simulink library "ECO_TestLibs"  (R2018a)
settings: Solver=ode45  StartTime=0.0  StopTime=10.0  RelTol=1e-3  EnableMultiTasking=on
undefined symbols (not defined in the file or in its folder): h, km
libraries: CoderSF_BSW_Libs x643, $bdroot x217, SF_CanService_Libs x60, simulink x12
(part 6 of 7)

== system ECO_TestLibs/LINASlave/Rx/Subsystem2 ==
  In1 : Inport
  Enable : EnablePort
  1 : Constant  Value=0  OutDataTypeStr=Inherit: Inherit via back propagation
  2 : Constant  Value=0  OutDataTypeStr=Inherit: Inherit via back propagation
  3 : Constant  Value=hex2dec('212')  OutDataTypeStr=Inherit: Inherit via back propagation
  4 : Constant  Value=8  OutDataTypeStr=Inherit: Inherit via back propagation
  Demux : Demux  Outputs=3
  Transmit CAN Message : CoderSF_BSW_Libs/CAN/Transmit CAN Message  channel=CAN_C  tasktimeIndex=Task_Inherit
      settings: SourceProductName=EcoCoder Blocks
  Vector Concatenate : Concatenate  NumInputs=8
  Write Measurement : CoderSF_BSW_Libs/Calibration & Measurement/Write Measurement  variable_name=LIN_Rx2  variable_value=0  variable_type=uint8  numD=3  unitStr=""  descStr=""
      settings: AttributesFormatString=type:%<variable_type> Dimensions:%<numD>  SourceProductName=EcoCoder Blocks
  cntValue : Subsystem
  wires:
  In1/1 -> Demux/1, Write Measurement/1
  3/1 -> Transmit CAN Message/3
  4/1 -> Transmit CAN Message/4
  2/1 -> Transmit CAN Message/2
  1/1 -> Transmit CAN Message/1
  Demux/2 -> Vector Concatenate/2
  Demux/1 -> Vector Concatenate/1
  Demux/3 -> Vector Concatenate/3
  Vector Concatenate/1 -> Transmit CAN Message/5
  cntValue/1(Out1) -> Vector Concatenate/4
  cntValue/2(Out2) -> Vector Concatenate/5
  cntValue/3(Out3) -> Vector Concatenate/6
  cntValue/4(Out4) -> Vector Concatenate/7
  cntValue/5(Out5) -> Vector Concatenate/8

== system ECO_TestLibs/LINASlave/Transmit/Tx ==
  Constant : Constant  OutDataTypeStr=uint8
  Constant1 : Constant  Value=2  OutDataTypeStr=uint8
  Data Type Conversion : DataTypeConversion
  Data Type Conversion1 : DataTypeConversion
  Delay : simulink/Discrete/Integer Delay  NumDelays=1  vinit=0  samptime=-1
      settings: SourceProductName=Simulink  SourceProductBaseCode=SL
  Delay1 : simulink/Discrete/Integer Delay  NumDelays=1  vinit=0  samptime=-1
      settings: SourceProductName=Simulink  SourceProductBaseCode=SL
  LIN Transmit Data2 : CoderSF_BSW_Libs/LIN/LIN Transmit Data  channel=LIN_A  Frame_Id=hex2dec('4')  Frame_Len=8  Frame_Dir=MasterReceive  Frame_CCS=Enhanced  Task_TimeIdx=Task_Inherit
      settings: SourceProductName=EcoCoder Blocks
  LIN Transmit Data3 : CoderSF_BSW_Libs/LIN/LIN Transmit Data  channel=LIN_A  Frame_Id=hex2dec('5')  Frame_Len=8  Frame_Dir=MasterReceive  Frame_CCS=Enhanced  Task_TimeIdx=Task_Inherit
      settings: SourceProductName=EcoCoder Blocks
  Mux : Mux  Inputs=8
  Mux1 : Mux  Inputs=8
  Sum : Sum  Inputs=|++
  Sum1 : Sum  Inputs=|++
  Write and Read Measurement : CoderSF_BSW_Libs/Calibration & Measurement/Write and Read Measurement  variable_name=LIN_ID4_SendData  variable_value=0  variable_type=uint8  numD=8  unitStr=""  descStr=""
      settings: AttributesFormatString=type:%<variable_type> Dimensions:%<numD>  SourceProductName=EcoCoder Blocks
  Write and Read Measurement1 : CoderSF_BSW_Libs/Calibration & Measurement/Write and Read Measurement  variable_name=LIN_ID5_SendData  variable_value=0  variable_type=uint8  numD=8  unitStr=""  descStr=""
      settings: AttributesFormatString=type:%<variable_type> Dimensions:%<numD>  SourceProductName=EcoCoder Blocks
  wires:
  Mux/1 -> Data Type Conversion/1
  Mux1/1 -> Data Type Conversion1/1
  Sum/1 -> Delay/1
  Constant/1 -> Sum/2
  Delay1/1 -> Sum1/1, Mux1/8, Mux1/7, Mux1/6, Mux1/5, Mux1/4, Mux1/3, Mux1/2, Mux1/1
  Sum1/1 -> Delay1/1
  Constant1/1 -> Sum1/2
  Write and Read Measurement/1 -> LIN Transmit Data2/1
  Data Type Conversion/1 -> Write and Read Measurement/1
  Delay/1 -> Mux/8, Mux/7, Mux/6, Mux/5, Mux/4, Mux/3, Mux/2, Mux/1, Sum/1
  Data Type Conversion1/1 -> Write and Read Measurement1/1
  Write and Read Measurement1/1 -> LIN Transmit Data3/1

== system ECO_TestLibs/TAF_CANA/Connected/Subsystem ==
  In1 : Inport
  In2 : Inport  Port=2
  In3 : Inport  Port=3
  In4 : Inport  Port=4
  In5 : Inport  Port=5
  In6 : Inport  Port=6
  In7 : Inport  Port=7
  In8 : Inport  Port=8
  Enable : EnablePort
  Plus1_{0..7} (8 alike) : $bdroot/Plus1_0
  Send Fixed-Point CAN Message : SF_CanService_Libs/Send Fixed-Point CAN Message  typeCAN=Connected  channel=CAN_A  mEn=off  msgInfo=TAF_CAN_new  msgIterm=CAN0x402  msgItermStore=CAN0x402  motoBit=off  flgNoFixed=off  tSample=Task_Inherit  modeCode=Parameterless
  wires:
  Plus1_4/1 -> Send Fixed-Point CAN Message/5
  Plus1_7/1 -> Send Fixed-Point CAN Message/8
  Plus1_6/1 -> Send Fixed-Point CAN Message/7
  Plus1_5/1 -> Send Fixed-Point CAN Message/6
  Plus1_3/1 -> Send Fixed-Point CAN Message/4
  Plus1_2/1 -> Send Fixed-Point CAN Message/3
  Plus1_1/1 -> Send Fixed-Point CAN Message/2
  Plus1_0/1 -> Send Fixed-Point CAN Message/1
  In7/1 -> Plus1_6/1
  In6/1 -> Plus1_5/1
  In8/1 -> Plus1_7/1
  In2/1 -> Plus1_1/1
  In3/1 -> Plus1_2/1
  In1/1 -> Plus1_0/1
  In5/1 -> Plus1_4/1
  In4/1 -> Plus1_3/1

== system ECO_TestLibs/TAF_CANA/Connected/Subsystem1 ==
  In1 : Inport
  In2 : Inport  Port=2
  In3 : Inport  Port=3
  In4 : Inport  Port=4
  In5 : Inport  Port=5
  In6 : Inport  Port=6
  In7 : Inport  Port=7
  In8 : Inport  Port=8
  Enable : EnablePort
  Mux : Mux  Inputs=8
  Plus1_0 : $bdroot/Plus1_0
  Plus1_{1..7} (7 alike) : $bdroot/Plus2_0
  Plus2_0 : $bdroot/Plus2_0
  Send CAN Data : CoderSF_BSW_Libs/CAN/Send CAN Data  channel=CAN_A  txlen=8  txid=hex2dec('412')  frametype=Extended(29-bit ID)  showerror=off
      settings: SourceProductName=EcoCoder Blocks
  Send CAN Message : SF_CanService_Libs/Send CAN Message   typeCAN=Connected  channel=CAN_A  mEn=off  msgInfo=TAF_CAN_new  msgIterm=CAN0x402x  msgItermStore=CAN0x402x  motoBit=off  flgNoFixed=off  tSample=Task_Inherit  modeCode=Parameterless
  wires:
  Plus1_0/1 -> Send CAN Data/1
  Mux/1 -> Plus1_0/1
  In4/1 -> Plus1_3/1
  In5/1 -> Plus1_4/1
  In1/1 -> Plus2_0/1
  In3/1 -> Plus1_2/1
  In2/1 -> Plus1_1/1
  In8/1 -> Plus1_7/1
  In6/1 -> Plus1_5/1
  In7/1 -> Plus1_6/1
  Plus2_0/1 -> Send CAN Message/1, Mux/1
  Plus1_1/1 -> Send CAN Message/2, Mux/2
  Plus1_2/1 -> Send CAN Message/3, Mux/3
  Plus1_3/1 -> Send CAN Message/4, Mux/4
  Plus1_5/1 -> Send CAN Message/6, Mux/6
  Plus1_6/1 -> Send CAN Message/7, Mux/7
  Plus1_7/1 -> Send CAN Message/8, Mux/8
  Plus1_4/1 -> Send CAN Message/5, Mux/5

== system ECO_TestLibs/TAF_CANA/Disconnected/Subsystem ==
  In1 : Inport
  In2 : Inport  Port=2
  In3 : Inport  Port=3
  In4 : Inport  Port=4
  In5 : Inport  Port=5
  In6 : Inport  Port=6
  In7 : Inport  Port=7
  In8 : Inport  Port=8
  Enable : EnablePort
  Plus1_{0..7} (8 alike) : $bdroot/Plus1_0
  Send Fixed-Point CAN Message : SF_CanService_Libs/Send Fixed-Point CAN Message  typeCAN=Disconnected  channel=CAN_A  mEn=off  msgInfo=TAF_CAN_new  msgIterm=CAN0x401  msgItermStore=CAN0x401  motoBit=off  flgNoFixed=off  tSample=Task_Inherit  modeCode=Parameterless
  Transmit CAN Message : CoderSF_BSW_Libs/CAN/Transmit CAN Message  channel=CAN_A  tasktimeIndex=Task_Inherit
      settings: SourceProductName=EcoCoder Blocks
  wires:
  In4/1 -> Plus1_3/1
  In5/1 -> Plus1_4/1
  In1/1 -> Plus1_0/1
  In3/1 -> Plus1_2/1
  In2/1 -> Plus1_1/1
  In8/1 -> Plus1_7/1
  In6/1 -> Plus1_5/1
  In7/1 -> Plus1_6/1
  Plus1_0/1 -> Send Fixed-Point CAN Message/1
  Plus1_1/1 -> Send Fixed-Point CAN Message/2
  Plus1_2/1 -> Send Fixed-Point CAN Message/3
  Plus1_3/1 -> Send Fixed-Point CAN Message/4
  Plus1_5/1 -> Send Fixed-Point CAN Message/6
  Plus1_6/1 -> Send Fixed-Point CAN Message/7
  Plus1_7/1 -> Send Fixed-Point CAN Message/8
  Plus1_4/1 -> Send Fixed-Point CAN Message/5
  Send Fixed-Point CAN Message/4 -> Transmit CAN Message/4
  Send Fixed-Point CAN Message/5 -> Transmit CAN Message/5
  Send Fixed-Point CAN Message/1 -> Transmit CAN Message/1
  Send Fixed-Point CAN Message/2 -> Transmit CAN Message/2
  Send Fixed-Point CAN Message/3 -> Transmit CAN Message/3

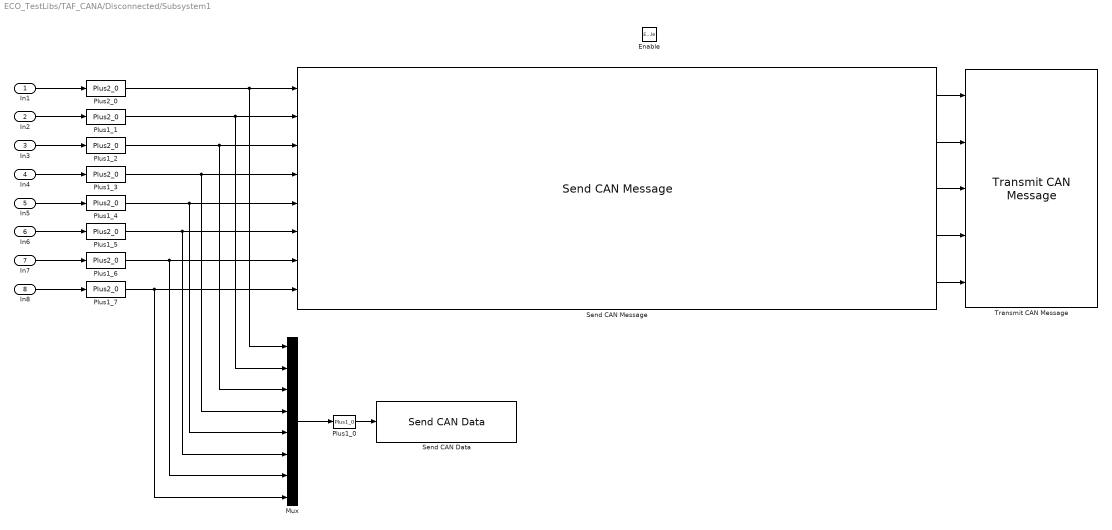
== system ECO_TestLibs/TAF_CANA/Disconnected/Subsystem1 ==
  In1 : Inport
  In2 : Inport  Port=2
  In3 : Inport  Port=3
  In4 : Inport  Port=4
  In5 : Inport  Port=5
  In6 : Inport  Port=6
  In7 : Inport  Port=7
  In8 : Inport  Port=8
  Enable : EnablePort
  Mux : Mux  Inputs=8
  Plus1_0 : $bdroot/Plus1_0
  Plus1_{1..7} (7 alike) : $bdroot/Plus2_0
  Plus2_0 : $bdroot/Plus2_0
  Send CAN Data : CoderSF_BSW_Libs/CAN/Send CAN Data  channel=CAN_A  txlen=8  txid=hex2dec('411')  frametype=Extended(29-bit ID)  showerror=off
      settings: SourceProductName=EcoCoder Blocks
  Send CAN Message : SF_CanService_Libs/Send CAN Message   typeCAN=Disconnected  channel=CAN_A  mEn=off  msgInfo=TAF_CAN_new  msgIterm=CAN0x401x  msgItermStore=CAN0x401x  motoBit=off  flgNoFixed=off  tSample=Task_Inherit  modeCode=Parameterless
  Transmit CAN Message : CoderSF_BSW_Libs/CAN/Transmit CAN Message  channel=CAN_A  tasktimeIndex=Task_Inherit
      settings: SourceProductName=EcoCoder Blocks
  wires:
  Plus1_4/1 -> Mux/5, Send CAN Message/5
  Plus1_7/1 -> Mux/8, Send CAN Message/8
  Plus1_6/1 -> Mux/7, Send CAN Message/7
  Plus1_5/1 -> Mux/6, Send CAN Message/6
  Plus1_3/1 -> Mux/4, Send CAN Message/4
  Plus1_2/1 -> Mux/3, Send CAN Message/3
  Plus1_1/1 -> Mux/2, Send CAN Message/2
  Plus2_0/1 -> Mux/1, Send CAN Message/1
  In7/1 -> Plus1_6/1
  In6/1 -> Plus1_5/1
  In8/1 -> Plus1_7/1
  In2/1 -> Plus1_1/1
  In3/1 -> Plus1_2/1
  In1/1 -> Plus2_0/1
  In5/1 -> Plus1_4/1
  In4/1 -> Plus1_3/1
  Mux/1 -> Plus1_0/1
  Plus1_0/1 -> Send CAN Data/1
  Send CAN Message/1 -> Transmit CAN Message/1
  Send CAN Message/5 -> Transmit CAN Message/5
  Send CAN Message/4 -> Transmit CAN Message/4
  Send CAN Message/2 -> Transmit CAN Message/2
  Send CAN Message/3 -> Transmit CAN Message/3

== system ECO_TestLibs/TAF_CANB/Connected/Subsystem1 ==
  In1 : Inport
  In2 : Inport  Port=2
  In3 : Inport  Port=3
  In4 : Inport  Port=4
  In5 : Inport  Port=5
  In6 : Inport  Port=6
  In7 : Inport  Port=7
  In8 : Inport  Port=8
  Enable : EnablePort
  Plus1_{0..7} (8 alike) : $bdroot/Plus1_0
  Send Fixed-Point CAN Message : SF_CanService_Libs/Send Fixed-Point CAN Message  typeCAN=Connected  channel=CAN_B  mEn=off  msgInfo=TAF_CAN_new  msgIterm=CAN0x404  msgItermStore=CAN0x404  motoBit=off  flgNoFixed=off  tSample=Task_Inherit  modeCode=Parameterless
  wires:
  Plus1_4/1 -> Send Fixed-Point CAN Message/5
  Plus1_7/1 -> Send Fixed-Point CAN Message/8
  Plus1_6/1 -> Send Fixed-Point CAN Message/7
  Plus1_5/1 -> Send Fixed-Point CAN Message/6
  Plus1_3/1 -> Send Fixed-Point CAN Message/4
  Plus1_2/1 -> Send Fixed-Point CAN Message/3
  Plus1_1/1 -> Send Fixed-Point CAN Message/2
  Plus1_0/1 -> Send Fixed-Point CAN Message/1
  In7/1 -> Plus1_6/1
  In6/1 -> Plus1_5/1
  In8/1 -> Plus1_7/1
  In2/1 -> Plus1_1/1
  In3/1 -> Plus1_2/1
  In1/1 -> Plus1_0/1
  In5/1 -> Plus1_4/1
  In4/1 -> Plus1_3/1

== system ECO_TestLibs/TAF_CANB/Connected/Subsystem5 ==
  In1 : Inport
  In2 : Inport  Port=2
  In3 : Inport  Port=3
  In4 : Inport  Port=4
  In5 : Inport  Port=5
  In6 : Inport  Port=6
  In7 : Inport  Port=7
  In8 : Inport  Port=8
  Enable : EnablePort
  Mux : Mux  Inputs=8
  Plus1_0 : $bdroot/Plus1_0
  Plus1_{1..7} (7 alike) : $bdroot/Plus2_0
  Plus2_0 : $bdroot/Plus2_0
  Send CAN Data : CoderSF_BSW_Libs/CAN/Send CAN Data  channel=CAN_B  txlen=8  txid=hex2dec('414')  frametype=Extended(29-bit ID)  showerror=off
      settings: SourceProductName=EcoCoder Blocks
  Send CAN Message : SF_CanService_Libs/Send CAN Message   typeCAN=Connected  channel=CAN_B  mEn=off  msgInfo=TAF_CAN_new  msgIterm=CAN0x404x  msgItermStore=CAN0x404x  motoBit=off  flgNoFixed=off  tSample=Task_Inherit  modeCode=Parameterless
  wires:
  Plus1_0/1 -> Send CAN Data/1
  Mux/1 -> Plus1_0/1
  In4/1 -> Plus1_3/1
  In5/1 -> Plus1_4/1
  In1/1 -> Plus2_0/1
  In3/1 -> Plus1_2/1
  In2/1 -> Plus1_1/1
  In8/1 -> Plus1_7/1
  In6/1 -> Plus1_5/1
  In7/1 -> Plus1_6/1
  Plus2_0/1 -> Send CAN Message/1, Mux/1
  Plus1_1/1 -> Send CAN Message/2, Mux/2
  Plus1_2/1 -> Send CAN Message/3, Mux/3
  Plus1_3/1 -> Send CAN Message/4, Mux/4
  Plus1_5/1 -> Send CAN Message/6, Mux/6
  Plus1_6/1 -> Send CAN Message/7, Mux/7
  Plus1_7/1 -> Send CAN Message/8, Mux/8
  Plus1_4/1 -> Send CAN Message/5, Mux/5

== system ECO_TestLibs/TAF_CANB/Disconnected/Subsystem1 ==
  In1 : Inport
  In2 : Inport  Port=2
  In3 : Inport  Port=3
  In4 : Inport  Port=4
  In5 : Inport  Port=5
  In6 : Inport  Port=6
  In7 : Inport  Port=7
  In8 : Inport  Port=8
  Enable : EnablePort
  Plus1_{0..7} (8 alike) : $bdroot/Plus1_0
  Send Fixed-Point CAN Message : SF_CanService_Libs/Send Fixed-Point CAN Message  typeCAN=Disconnected  channel=CAN_B  mEn=off  msgInfo=TAF_CAN_new  msgIterm=CAN0x403  msgItermStore=CAN0x403  motoBit=off  flgNoFixed=off  tSample=Task_Inherit  modeCode=Parameterless
  Transmit CAN Message : CoderSF_BSW_Libs/CAN/Transmit CAN Message  channel=CAN_B  tasktimeIndex=Task_Inherit
      settings: SourceProductName=EcoCoder Blocks
  wires:
  In4/1 -> Plus1_3/1
  In5/1 -> Plus1_4/1
  In1/1 -> Plus1_0/1
  In3/1 -> Plus1_2/1
  In2/1 -> Plus1_1/1
  In8/1 -> Plus1_7/1
  In6/1 -> Plus1_5/1
  In7/1 -> Plus1_6/1
  Plus1_0/1 -> Send Fixed-Point CAN Message/1
  Plus1_1/1 -> Send Fixed-Point CAN Message/2
  Plus1_2/1 -> Send Fixed-Point CAN Message/3
  Plus1_3/1 -> Send Fixed-Point CAN Message/4
  Plus1_5/1 -> Send Fixed-Point CAN Message/6
  Plus1_6/1 -> Send Fixed-Point CAN Message/7
  Plus1_7/1 -> Send Fixed-Point CAN Message/8
  Plus1_4/1 -> Send Fixed-Point CAN Message/5
  Send Fixed-Point CAN Message/3 -> Transmit CAN Message/3
  Send Fixed-Point CAN Message/4 -> Transmit CAN Message/4
  Send Fixed-Point CAN Message/2 -> Transmit CAN Message/2
  Send Fixed-Point CAN Message/1 -> Transmit CAN Message/1
  Send Fixed-Point CAN Message/5 -> Transmit CAN Message/5

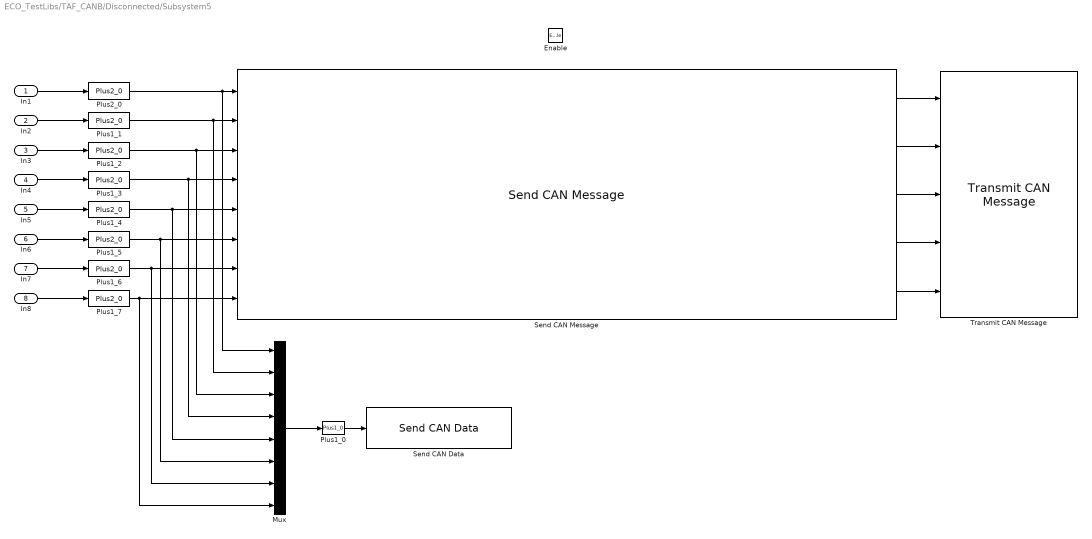
== system ECO_TestLibs/TAF_CANB/Disconnected/Subsystem5 ==
  In1 : Inport
  In2 : Inport  Port=2
  In3 : Inport  Port=3
  In4 : Inport  Port=4
  In5 : Inport  Port=5
  In6 : Inport  Port=6
  In7 : Inport  Port=7
  In8 : Inport  Port=8
  Enable : EnablePort
  Mux : Mux  Inputs=8
  Plus1_0 : $bdroot/Plus1_0
  Plus1_{1..7} (7 alike) : $bdroot/Plus2_0
  Plus2_0 : $bdroot/Plus2_0
  Send CAN Data : CoderSF_BSW_Libs/CAN/Send CAN Data  channel=CAN_B  txlen=8  txid=hex2dec('413')  frametype=Extended(29-bit ID)  showerror=off
      settings: SourceProductName=EcoCoder Blocks
  Send CAN Message : SF_CanService_Libs/Send CAN Message   typeCAN=Disconnected  channel=CAN_B  mEn=off  msgInfo=TAF_CAN_new  msgIterm=CAN0x403x  msgItermStore=CAN0x403x  motoBit=off  flgNoFixed=off  tSample=Task_Inherit  modeCode=Parameterless
  Transmit CAN Message : CoderSF_BSW_Libs/CAN/Transmit CAN Message  channel=CAN_B  tasktimeIndex=Task_Inherit
      settings: SourceProductName=EcoCoder Blocks
  wires:
  Plus1_4/1 -> Mux/5, Send CAN Message/5
  Plus1_7/1 -> Mux/8, Send CAN Message/8
  Plus1_6/1 -> Mux/7, Send CAN Message/7
  Plus1_5/1 -> Mux/6, Send CAN Message/6
  Plus1_3/1 -> Mux/4, Send CAN Message/4
  Plus1_2/1 -> Mux/3, Send CAN Message/3
  Plus1_1/1 -> Mux/2, Send CAN Message/2
  Plus2_0/1 -> Mux/1, Send CAN Message/1
  In7/1 -> Plus1_6/1
  In6/1 -> Plus1_5/1
  In8/1 -> Plus1_7/1
  In2/1 -> Plus1_1/1
  In3/1 -> Plus1_2/1
  In1/1 -> Plus2_0/1
  In5/1 -> Plus1_4/1
  In4/1 -> Plus1_3/1
  Mux/1 -> Plus1_0/1
  Plus1_0/1 -> Send CAN Data/1
  Send CAN Message/3 -> Transmit CAN Message/3
  Send CAN Message/2 -> Transmit CAN Message/2
  Send CAN Message/4 -> Transmit CAN Message/4
  Send CAN Message/5 -> Transmit CAN Message/5
  Send CAN Message/1 -> Transmit CAN Message/1

== system ECO_TestLibs/TAF_CANC/Connected/Subsystem2 ==
  In1 : Inport
  In2 : Inport  Port=2
  In3 : Inport  Port=3
  In4 : Inport  Port=4
  In5 : Inport  Port=5
  In6 : Inport  Port=6
  In7 : Inport  Port=7
  In8 : Inport  Port=8
  Enable : EnablePort
  Plus1_{0..7} (8 alike) : $bdroot/Plus1_0
  Send Fixed-Point CAN Message : SF_CanService_Libs/Send Fixed-Point CAN Message  typeCAN=Connected  channel=CAN_C  mEn=off  msgInfo=TAF_CAN_new  msgIterm=CAN0x406  msgItermStore=CAN0x406  motoBit=off  flgNoFixed=off  tSample=Task_Inherit  modeCode=Parameterless
  wires:
  In4/1 -> Plus1_3/1
  In5/1 -> Plus1_4/1
  In1/1 -> Plus1_0/1
  In3/1 -> Plus1_2/1
  In2/1 -> Plus1_1/1
  In8/1 -> Plus1_7/1
  In6/1 -> Plus1_5/1
  In7/1 -> Plus1_6/1
  Plus1_0/1 -> Send Fixed-Point CAN Message/1
  Plus1_1/1 -> Send Fixed-Point CAN Message/2
  Plus1_2/1 -> Send Fixed-Point CAN Message/3
  Plus1_3/1 -> Send Fixed-Point CAN Message/4
  Plus1_5/1 -> Send Fixed-Point CAN Message/6
  Plus1_6/1 -> Send Fixed-Point CAN Message/7
  Plus1_7/1 -> Send Fixed-Point CAN Message/8
  Plus1_4/1 -> Send Fixed-Point CAN Message/5

== system ECO_TestLibs/TAF_CANC/Connected/Subsystem6 ==
  In1 : Inport
  In2 : Inport  Port=2
  In3 : Inport  Port=3
  In4 : Inport  Port=4
  In5 : Inport  Port=5
  In6 : Inport  Port=6
  In7 : Inport  Port=7
  In8 : Inport  Port=8
  Enable : EnablePort
  Mux : Mux  Inputs=8
  Plus1_0 : $bdroot/Plus1_0
  Plus1_{1..7} (7 alike) : $bdroot/Plus2_0
  Plus2_0 : $bdroot/Plus2_0
  Send CAN Data : CoderSF_BSW_Libs/CAN/Send CAN Data  channel=CAN_C  txlen=8  txid=hex2dec('416')  frametype=Extended(29-bit ID)  showerror=off
      settings: SourceProductName=EcoCoder Blocks
  Send CAN Message : SF_CanService_Libs/Send CAN Message   typeCAN=Connected  channel=CAN_C  mEn=off  msgInfo=TAF_CAN_new  msgIterm=CAN0x406x  msgItermStore=CAN0x406x  motoBit=off  flgNoFixed=off  tSample=Task_Inherit  modeCode=Parameterless
  wires:
  In7/1 -> Plus1_6/1
  In6/1 -> Plus1_5/1
  In8/1 -> Plus1_7/1
  In2/1 -> Plus1_1/1
  In3/1 -> Plus1_2/1
  In1/1 -> Plus2_0/1
  In5/1 -> Plus1_4/1
  In4/1 -> Plus1_3/1
  Plus1_4/1 -> Mux/5, Send CAN Message/5
  Plus1_7/1 -> Mux/8, Send CAN Message/8
  Plus1_6/1 -> Mux/7, Send CAN Message/7
  Plus1_5/1 -> Mux/6, Send CAN Message/6
  Plus1_3/1 -> Mux/4, Send CAN Message/4
  Plus1_2/1 -> Mux/3, Send CAN Message/3
  Plus1_1/1 -> Mux/2, Send CAN Message/2
  Plus2_0/1 -> Mux/1, Send CAN Message/1
  Mux/1 -> Plus1_0/1
  Plus1_0/1 -> Send CAN Data/1

== system ECO_TestLibs/TAF_CANC/Disconnected/Subsystem2 ==
  In1 : Inport
  In2 : Inport  Port=2
  In3 : Inport  Port=3
  In4 : Inport  Port=4
  In5 : Inport  Port=5
  In6 : Inport  Port=6
  In7 : Inport  Port=7
  In8 : Inport  Port=8
  Enable : EnablePort
  Plus1_{0..7} (8 alike) : $bdroot/Plus1_0
  Send Fixed-Point CAN Message : SF_CanService_Libs/Send Fixed-Point CAN Message  typeCAN=Disconnected  channel=CAN_C  mEn=off  msgInfo=TAF_CAN_new  msgIterm=CAN0x405  msgItermStore=CAN0x405  motoBit=off  flgNoFixed=off  tSample=Task_Inherit  modeCode=Parameterless
  Transmit CAN Message : CoderSF_BSW_Libs/CAN/Transmit CAN Message  channel=CAN_C  tasktimeIndex=Task_Inherit
      settings: SourceProductName=EcoCoder Blocks
  wires:
  Plus1_4/1 -> Send Fixed-Point CAN Message/5
  Plus1_7/1 -> Send Fixed-Point CAN Message/8
  Plus1_6/1 -> Send Fixed-Point CAN Message/7
  Plus1_5/1 -> Send Fixed-Point CAN Message/6
  Plus1_3/1 -> Send Fixed-Point CAN Message/4
  Plus1_2/1 -> Send Fixed-Point CAN Message/3
  Plus1_1/1 -> Send Fixed-Point CAN Message/2
  Plus1_0/1 -> Send Fixed-Point CAN Message/1
  In7/1 -> Plus1_6/1
  In6/1 -> Plus1_5/1
  In8/1 -> Plus1_7/1
  In2/1 -> Plus1_1/1
  In3/1 -> Plus1_2/1
  In1/1 -> Plus1_0/1
  In5/1 -> Plus1_4/1
  In4/1 -> Plus1_3/1
  Send Fixed-Point CAN Message/3 -> Transmit CAN Message/3
  Send Fixed-Point CAN Message/1 -> Transmit CAN Message/1
  Send Fixed-Point CAN Message/2 -> Transmit CAN Message/2
  Send Fixed-Point CAN Message/5 -> Transmit CAN Message/5
  Send Fixed-Point CAN Message/4 -> Transmit CAN Message/4

== system ECO_TestLibs/TAF_CANC/Disconnected/Subsystem6 ==
  In1 : Inport
  In2 : Inport  Port=2
  In3 : Inport  Port=3
  In4 : Inport  Port=4
  In5 : Inport  Port=5
  In6 : Inport  Port=6
  In7 : Inport  Port=7
  In8 : Inport  Port=8
  Enable : EnablePort
  Mux : Mux  Inputs=8
  Plus1_0 : $bdroot/Plus1_0
  Plus1_{1..7} (7 alike) : $bdroot/Plus2_0
  Plus2_0 : $bdroot/Plus2_0
  Send CAN Data : CoderSF_BSW_Libs/CAN/Send CAN Data  channel=CAN_C  txlen=8  txid=hex2dec('415')  frametype=Extended(29-bit ID)  showerror=off
      settings: SourceProductName=EcoCoder Blocks
  Send CAN Message : SF_CanService_Libs/Send CAN Message   typeCAN=Disconnected  channel=CAN_C  mEn=off  msgInfo=TAF_CAN_new  msgIterm=CAN0x405x  msgItermStore=CAN0x405x  motoBit=off  flgNoFixed=off  tSample=Task_Inherit  modeCode=Parameterless
  Transmit CAN Message : CoderSF_BSW_Libs/CAN/Transmit CAN Message  channel=CAN_C  tasktimeIndex=Task_Inherit
      settings: SourceProductName=EcoCoder Blocks
  wires:
  Plus1_0/1 -> Send CAN Data/1
  Mux/1 -> Plus1_0/1
  Plus2_0/1 -> Send CAN Message/1, Mux/1
  Plus1_1/1 -> Send CAN Message/2, Mux/2
  Plus1_2/1 -> Send CAN Message/3, Mux/3
  Plus1_3/1 -> Send CAN Message/4, Mux/4
  Plus1_5/1 -> Send CAN Message/6, Mux/6
  Plus1_6/1 -> Send CAN Message/7, Mux/7
  Plus1_7/1 -> Send CAN Message/8, Mux/8
  Plus1_4/1 -> Send CAN Message/5, Mux/5
  In4/1 -> Plus1_3/1
  In5/1 -> Plus1_4/1
  In1/1 -> Plus2_0/1
  In3/1 -> Plus1_2/1
  In2/1 -> Plus1_1/1
  In8/1 -> Plus1_7/1
  In6/1 -> Plus1_5/1
  In7/1 -> Plus1_6/1
  Send CAN Message/5 -> Transmit CAN Message/5
  Send CAN Message/2 -> Transmit CAN Message/2
  Send CAN Message/3 -> Transmit CAN Message/3
  Send CAN Message/4 -> Transmit CAN Message/4
  Send CAN Message/1 -> Transmit CAN Message/1

== system ECO_TestLibs/TAF_CAND/Connected/Subsystem3 ==
  In1 : Inport
  In2 : Inport  Port=2
  In3 : Inport  Port=3
  In4 : Inport  Port=4
  In5 : Inport  Port=5
  In6 : Inport  Port=6
  In7 : Inport  Port=7
  In8 : Inport  Port=8
  Enable : EnablePort
  Plus1_{0..7} (8 alike) : $bdroot/Plus1_0
  Send Fixed-Point CAN Message : SF_CanService_Libs/Send Fixed-Point CAN Message  typeCAN=Connected  channel=CAN_D  mEn=off  msgInfo=TAF_CAN_new  msgIterm=CAN0x408  msgItermStore=CAN0x408  motoBit=off  flgNoFixed=off  tSample=Task_Inherit  modeCode=Parameterless
  wires:
  Plus1_4/1 -> Send Fixed-Point CAN Message/5
  Plus1_7/1 -> Send Fixed-Point CAN Message/8
  Plus1_6/1 -> Send Fixed-Point CAN Message/7
  Plus1_5/1 -> Send Fixed-Point CAN Message/6
  Plus1_3/1 -> Send Fixed-Point CAN Message/4
  Plus1_2/1 -> Send Fixed-Point CAN Message/3
  Plus1_1/1 -> Send Fixed-Point CAN Message/2
  Plus1_0/1 -> Send Fixed-Point CAN Message/1
  In7/1 -> Plus1_6/1
  In6/1 -> Plus1_5/1
  In8/1 -> Plus1_7/1
  In2/1 -> Plus1_1/1
  In3/1 -> Plus1_2/1
  In1/1 -> Plus1_0/1
  In5/1 -> Plus1_4/1
  In4/1 -> Plus1_3/1

== system ECO_TestLibs/TAF_CAND/Connected/Subsystem7 ==
  In1 : Inport
  In2 : Inport  Port=2
  In3 : Inport  Port=3
  In4 : Inport  Port=4
  In5 : Inport  Port=5
  In6 : Inport  Port=6
  In7 : Inport  Port=7
  In8 : Inport  Port=8
  Enable : EnablePort
  Mux : Mux  Inputs=8
  Plus1_0 : $bdroot/Plus1_0
  Plus1_{1..7} (7 alike) : $bdroot/Plus2_0
  Plus2_0 : $bdroot/Plus2_0
  Send CAN Data : CoderSF_BSW_Libs/CAN/Send CAN Data  channel=CAN_D  txlen=8  txid=hex2dec('418')  frametype=Extended(29-bit ID)  showerror=off
      settings: SourceProductName=EcoCoder Blocks
  Send CAN Message : SF_CanService_Libs/Send CAN Message   typeCAN=Connected  channel=CAN_D  mEn=off  msgInfo=TAF_CAN_new  msgIterm=CAN0x408x  msgItermStore=CAN0x408x  motoBit=off  flgNoFixed=off  tSample=Task_Inherit  modeCode=Parameterless
  wires:
  Plus1_0/1 -> Send CAN Data/1
  Mux/1 -> Plus1_0/1
  Plus2_0/1 -> Send CAN Message/1, Mux/1
  Plus1_1/1 -> Send CAN Message/2, Mux/2
  Plus1_2/1 -> Send CAN Message/3, Mux/3
  Plus1_3/1 -> Send CAN Message/4, Mux/4
  Plus1_5/1 -> Send CAN Message/6, Mux/6
  Plus1_6/1 -> Send CAN Message/7, Mux/7
  Plus1_7/1 -> Send CAN Message/8, Mux/8
  Plus1_4/1 -> Send CAN Message/5, Mux/5
  In4/1 -> Plus1_3/1
  In5/1 -> Plus1_4/1
  In1/1 -> Plus2_0/1
  In3/1 -> Plus1_2/1
  In2/1 -> Plus1_1/1
  In8/1 -> Plus1_7/1
  In6/1 -> Plus1_5/1
  In7/1 -> Plus1_6/1

== system ECO_TestLibs/TAF_CAND/Disconnected/Subsystem3 ==
  In1 : Inport
  In2 : Inport  Port=2
  In3 : Inport  Port=3
  In4 : Inport  Port=4
  In5 : Inport  Port=5
  In6 : Inport  Port=6
  In7 : Inport  Port=7
  In8 : Inport  Port=8
  Enable : EnablePort
  Plus1_{0..7} (8 alike) : $bdroot/Plus1_0
  Send Fixed-Point CAN Message : SF_CanService_Libs/Send Fixed-Point CAN Message  typeCAN=Disconnected  channel=CAN_D  mEn=off  msgInfo=TAF_CAN_new  msgIterm=CAN0x407  msgItermStore=CAN0x407  motoBit=off  flgNoFixed=off  tSample=Task_Inherit  modeCode=Parameterless
  Transmit CAN Message : CoderSF_BSW_Libs/CAN/Transmit CAN Message  channel=CAN_D  tasktimeIndex=Task_Inherit
      settings: SourceProductName=EcoCoder Blocks
  wires:
  In4/1 -> Plus1_3/1
  In5/1 -> Plus1_4/1
  In1/1 -> Plus1_0/1
  In3/1 -> Plus1_2/1
  In2/1 -> Plus1_1/1
  In8/1 -> Plus1_7/1
  In6/1 -> Plus1_5/1
  In7/1 -> Plus1_6/1
  Plus1_0/1 -> Send Fixed-Point CAN Message/1
  Plus1_1/1 -> Send Fixed-Point CAN Message/2
  Plus1_2/1 -> Send Fixed-Point CAN Message/3
  Plus1_3/1 -> Send Fixed-Point CAN Message/4
  Plus1_5/1 -> Send Fixed-Point CAN Message/6
  Plus1_6/1 -> Send Fixed-Point CAN Message/7
  Plus1_7/1 -> Send Fixed-Point CAN Message/8
  Plus1_4/1 -> Send Fixed-Point CAN Message/5
  Send Fixed-Point CAN Message/2 -> Transmit CAN Message/2
  Send Fixed-Point CAN Message/4 -> Transmit CAN Message/4
  Send Fixed-Point CAN Message/3 -> Transmit CAN Message/3
  Send Fixed-Point CAN Message/1 -> Transmit CAN Message/1
  Send Fixed-Point CAN Message/5 -> Transmit CAN Message/5

== system ECO_TestLibs/TAF_CAND/Disconnected/Subsystem7 ==
  In1 : Inport
  In2 : Inport  Port=2
  In3 : Inport  Port=3
  In4 : Inport  Port=4
  In5 : Inport  Port=5
  In6 : Inport  Port=6
  In7 : Inport  Port=7
  In8 : Inport  Port=8
  Enable : EnablePort
  Mux : Mux  Inputs=8
  Plus1_0 : $bdroot/Plus1_0
  Plus1_{1..7} (7 alike) : $bdroot/Plus2_0
  Plus2_0 : $bdroot/Plus2_0
  Send CAN Data : CoderSF_BSW_Libs/CAN/Send CAN Data  channel=CAN_D  txlen=8  txid=hex2dec('417')  frametype=Extended(29-bit ID)  showerror=off
      settings: SourceProductName=EcoCoder Blocks
  Send CAN Message : SF_CanService_Libs/Send CAN Message   typeCAN=Disconnected  channel=CAN_D  mEn=off  msgInfo=TAF_CAN_new  msgIterm=CAN0x407x  msgItermStore=CAN0x407x  motoBit=off  flgNoFixed=off  tSample=Task_Inherit  modeCode=Parameterless
  Transmit CAN Message : CoderSF_BSW_Libs/CAN/Transmit CAN Message  channel=CAN_D  tasktimeIndex=Task_Inherit
      settings: SourceProductName=EcoCoder Blocks
  wires:
  In7/1 -> Plus1_6/1
  In6/1 -> Plus1_5/1
  In8/1 -> Plus1_7/1
  In2/1 -> Plus1_1/1
  In3/1 -> Plus1_2/1
  In1/1 -> Plus2_0/1
  In5/1 -> Plus1_4/1
  In4/1 -> Plus1_3/1
  Plus1_4/1 -> Mux/5, Send CAN Message/5
  Plus1_7/1 -> Mux/8, Send CAN Message/8
  Plus1_6/1 -> Mux/7, Send CAN Message/7
  Plus1_5/1 -> Mux/6, Send CAN Message/6
  Plus1_3/1 -> Mux/4, Send CAN Message/4
  Plus1_2/1 -> Mux/3, Send CAN Message/3
  Plus1_1/1 -> Mux/2, Send CAN Message/2
  Plus2_0/1 -> Mux/1, Send CAN Message/1
  Mux/1 -> Plus1_0/1
  Plus1_0/1 -> Send CAN Data/1
  Send CAN Message/1 -> Transmit CAN Message/1
  Send CAN Message/2 -> Transmit CAN Message/2
  Send CAN Message/3 -> Transmit CAN Message/3
  Send CAN Message/4 -> Transmit CAN Message/4
  Send CAN Message/5 -> Transmit CAN Message/5

== system ECO_TestLibs/TAF_CANE/Connected/Subsystem4 ==
  In1 : Inport
  In2 : Inport  Port=2
  In3 : Inport  Port=3
  In4 : Inport  Port=4
  In5 : Inport  Port=5
  In6 : Inport  Port=6
  In7 : Inport  Port=7
  In8 : Inport  Port=8
  Enable : EnablePort
  Plus1_{0..7} (8 alike) : $bdroot/Plus1_0
  Send Fixed-Point CAN Message : SF_CanService_Libs/Send Fixed-Point CAN Message  typeCAN=Connected  channel=CAN_E  mEn=off  msgInfo=TAF_CAN_new  msgIterm=CAN0x410  msgItermStore=CAN0x410  motoBit=off  flgNoFixed=off  tSample=Task_Inherit  modeCode=Parameterless
  wires:
  In4/1 -> Plus1_3/1
  In5/1 -> Plus1_4/1
  In1/1 -> Plus1_0/1
  In3/1 -> Plus1_2/1
  In2/1 -> Plus1_1/1
  In8/1 -> Plus1_7/1
  In6/1 -> Plus1_5/1
  In7/1 -> Plus1_6/1
  Plus1_0/1 -> Send Fixed-Point CAN Message/1
  Plus1_1/1 -> Send Fixed-Point CAN Message/2
  Plus1_2/1 -> Send Fixed-Point CAN Message/3
  Plus1_3/1 -> Send Fixed-Point CAN Message/4
  Plus1_5/1 -> Send Fixed-Point CAN Message/6
  Plus1_6/1 -> Send Fixed-Point CAN Message/7
  Plus1_7/1 -> Send Fixed-Point CAN Message/8
  Plus1_4/1 -> Send Fixed-Point CAN Message/5

== system ECO_TestLibs/TAF_CANE/Connected/Subsystem8 ==
  In1 : Inport
  In2 : Inport  Port=2
  In3 : Inport  Port=3
  In4 : Inport  Port=4
  In5 : Inport  Port=5
  In6 : Inport  Port=6
  In7 : Inport  Port=7
  In8 : Inport  Port=8
  Enable : EnablePort
  Mux : Mux  Inputs=8
  Plus1_0 : $bdroot/Plus1_0
  Plus1_{1..7} (7 alike) : $bdroot/Plus2_0
  Plus2_0 : $bdroot/Plus2_0
  Send CAN Data : CoderSF_BSW_Libs/CAN/Send CAN Data  channel=CAN_E  txlen=8  txid=hex2dec('420')  frametype=Extended(29-bit ID)  showerror=off
      settings: SourceProductName=EcoCoder Blocks
  Send CAN Message : SF_CanService_Libs/Send CAN Message   typeCAN=Connected  channel=CAN_E  mEn=off  msgInfo=TAF_CAN_new  msgIterm=CAN0x410x  msgItermStore=CAN0x410x  motoBit=off  flgNoFixed=off  tSample=Task_Inherit  modeCode=Parameterless
  wires:
  In7/1 -> Plus1_6/1
  In6/1 -> Plus1_5/1
  In8/1 -> Plus1_7/1
  In2/1 -> Plus1_1/1
  In3/1 -> Plus1_2/1
  In1/1 -> Plus2_0/1
  In5/1 -> Plus1_4/1
  In4/1 -> Plus1_3/1
  Plus1_4/1 -> Mux/5, Send CAN Message/5
  Plus1_7/1 -> Mux/8, Send CAN Message/8
  Plus1_6/1 -> Mux/7, Send CAN Message/7
  Plus1_5/1 -> Mux/6, Send CAN Message/6
  Plus1_3/1 -> Mux/4, Send CAN Message/4
  Plus1_2/1 -> Mux/3, Send CAN Message/3
  Plus1_1/1 -> Mux/2, Send CAN Message/2
  Plus2_0/1 -> Mux/1, Send CAN Message/1
  Mux/1 -> Plus1_0/1
  Plus1_0/1 -> Send CAN Data/1

== system ECO_TestLibs/TAF_CANE/Disconnected/Subsystem4 ==
  In1 : Inport
  In2 : Inport  Port=2
  In3 : Inport  Port=3
  In4 : Inport  Port=4
  In5 : Inport  Port=5
  In6 : Inport  Port=6
  In7 : Inport  Port=7
  In8 : Inport  Port=8
  Enable : EnablePort
  Plus1_{0..7} (8 alike) : $bdroot/Plus1_0
  Send Fixed-Point CAN Message : SF_CanService_Libs/Send Fixed-Point CAN Message  typeCAN=Disconnected  channel=CAN_E  mEn=off  msgInfo=TAF_CAN_new  msgIterm=CAN0x409  msgItermStore=CAN0x409  motoBit=off  flgNoFixed=off  tSample=Task_Inherit  modeCode=Parameterless
  Transmit CAN Message : CoderSF_BSW_Libs/CAN/Transmit CAN Message  channel=CAN_E  tasktimeIndex=Task_Inherit
      settings: SourceProductName=EcoCoder Blocks
  wires:
  Send Fixed-Point CAN Message/4 -> Transmit CAN Message/4
  Send Fixed-Point CAN Message/3 -> Transmit CAN Message/3
  Send Fixed-Point CAN Message/5 -> Transmit CAN Message/5
  Send Fixed-Point CAN Message/1 -> Transmit CAN Message/1
  Send Fixed-Point CAN Message/2 -> Transmit CAN Message/2
  Plus1_4/1 -> Send Fixed-Point CAN Message/5
  Plus1_7/1 -> Send Fixed-Point CAN Message/8
  Plus1_6/1 -> Send Fixed-Point CAN Message/7
  Plus1_5/1 -> Send Fixed-Point CAN Message/6
  Plus1_3/1 -> Send Fixed-Point CAN Message/4
  Plus1_2/1 -> Send Fixed-Point CAN Message/3
  Plus1_1/1 -> Send Fixed-Point CAN Message/2
  Plus1_0/1 -> Send Fixed-Point CAN Message/1
  In7/1 -> Plus1_6/1
  In6/1 -> Plus1_5/1
  In8/1 -> Plus1_7/1
  In2/1 -> Plus1_1/1
  In3/1 -> Plus1_2/1
  In1/1 -> Plus1_0/1
  In5/1 -> Plus1_4/1
  In4/1 -> Plus1_3/1

== system ECO_TestLibs/TAF_CANE/Disconnected/Subsystem8 ==
  In1 : Inport
  In2 : Inport  Port=2
  In3 : Inport  Port=3
  In4 : Inport  Port=4
  In5 : Inport  Port=5
  In6 : Inport  Port=6
  In7 : Inport  Port=7
  In8 : Inport  Port=8
  Enable : EnablePort
  Mux : Mux  Inputs=8
  Plus1_0 : $bdroot/Plus1_0
  Plus1_{1..7} (7 alike) : $bdroot/Plus2_0
  Plus2_0 : $bdroot/Plus2_0
  Send CAN Data : CoderSF_BSW_Libs/CAN/Send CAN Data  channel=CAN_E  txlen=8  txid=hex2dec('419')  frametype=Extended(29-bit ID)  showerror=off
      settings: SourceProductName=EcoCoder Blocks
  Send CAN Message : SF_CanService_Libs/Send CAN Message   typeCAN=Disconnected  channel=CAN_E  mEn=off  msgInfo=TAF_CAN_new  msgIterm=CAN0x409x  msgItermStore=CAN0x409x  motoBit=off  flgNoFixed=off  tSample=Task_Inherit  modeCode=Parameterless
  Transmit CAN Message : CoderSF_BSW_Libs/CAN/Transmit CAN Message  channel=CAN_E  tasktimeIndex=Task_Inherit
      settings: SourceProductName=EcoCoder Blocks
  wires:
  Send CAN Message/3 -> Transmit CAN Message/3
  Send CAN Message/2 -> Transmit CAN Message/2
  Send CAN Message/4 -> Transmit CAN Message/4
  Send CAN Message/1 -> Transmit CAN Message/1
  Send CAN Message/5 -> Transmit CAN Message/5
  Plus1_0/1 -> Send CAN Data/1
  Mux/1 -> Plus1_0/1
  Plus2_0/1 -> Send CAN Message/1, Mux/1
  Plus1_1/1 -> Send CAN Message/2, Mux/2
  Plus1_2/1 -> Send CAN Message/3, Mux/3
  Plus1_3/1 -> Send CAN Message/4, Mux/4
  Plus1_5/1 -> Send CAN Message/6, Mux/6
  Plus1_6/1 -> Send CAN Message/7, Mux/7
  Plus1_7/1 -> Send CAN Message/8, Mux/8
  Plus1_4/1 -> Send CAN Message/5, Mux/5
  In4/1 -> Plus1_3/1
  In5/1 -> Plus1_4/1
  In1/1 -> Plus2_0/1
  In3/1 -> Plus1_2/1
  In2/1 -> Plus1_1/1
  In8/1 -> Plus1_7/1
  In6/1 -> Plus1_5/1
  In7/1 -> Plus1_6/1

== system ECO_TestLibs/TAF_CANF/Connected/Subsystem4 ==
  In1 : Inport
  In2 : Inport  Port=2
  In3 : Inport  Port=3
  In4 : Inport  Port=4
  In5 : Inport  Port=5
  In6 : Inport  Port=6
  In7 : Inport  Port=7
  In8 : Inport  Port=8
  Enable : EnablePort
  Plus1_{0..7} (8 alike) : $bdroot/Plus1_0
  Send Fixed-Point CAN Message : SF_CanService_Libs/Send Fixed-Point CAN Message  typeCAN=Connected  channel=CAN_F  mEn=off  msgInfo=TAF_CAN_new  msgIterm=CAN0x410  msgItermStore=CAN0x410  motoBit=off  flgNoFixed=off  tSample=Task_Inherit  modeCode=Parameterless
  wires:
  Plus1_4/1 -> Send Fixed-Point CAN Message/5
  Plus1_7/1 -> Send Fixed-Point CAN Message/8
  Plus1_6/1 -> Send Fixed-Point CAN Message/7
  Plus1_5/1 -> Send Fixed-Point CAN Message/6
  Plus1_3/1 -> Send Fixed-Point CAN Message/4
  Plus1_2/1 -> Send Fixed-Point CAN Message/3
  Plus1_1/1 -> Send Fixed-Point CAN Message/2
  Plus1_0/1 -> Send Fixed-Point CAN Message/1
  In7/1 -> Plus1_6/1
  In6/1 -> Plus1_5/1
  In8/1 -> Plus1_7/1
  In2/1 -> Plus1_1/1
  In3/1 -> Plus1_2/1
  In1/1 -> Plus1_0/1
  In5/1 -> Plus1_4/1
  In4/1 -> Plus1_3/1

== system ECO_TestLibs/TAF_CANF/Connected/Subsystem8 ==
  In1 : Inport
  In2 : Inport  Port=2
  In3 : Inport  Port=3
  In4 : Inport  Port=4
  In5 : Inport  Port=5
  In6 : Inport  Port=6
  In7 : Inport  Port=7
  In8 : Inport  Port=8
  Enable : EnablePort
  Mux : Mux  Inputs=8
  Plus1_0 : $bdroot/Plus1_0
  Plus1_{1..7} (7 alike) : $bdroot/Plus2_0
  Plus2_0 : $bdroot/Plus2_0
  Send CAN Data : CoderSF_BSW_Libs/CAN/Send CAN Data  channel=CAN_F  txlen=8  txid=hex2dec('420')  frametype=Extended(29-bit ID)  showerror=off
      settings: SourceProductName=EcoCoder Blocks
  Send CAN Message : SF_CanService_Libs/Send CAN Message   typeCAN=Connected  channel=CAN_F  mEn=off  msgInfo=TAF_CAN_new  msgIterm=CAN0x410x  msgItermStore=CAN0x410x  motoBit=off  flgNoFixed=off  tSample=Task_Inherit  modeCode=Parameterless
  wires:
  Plus1_0/1 -> Send CAN Data/1
  Mux/1 -> Plus1_0/1
  Plus2_0/1 -> Send CAN Message/1, Mux/1
  Plus1_1/1 -> Send CAN Message/2, Mux/2
  Plus1_2/1 -> Send CAN Message/3, Mux/3
  Plus1_3/1 -> Send CAN Message/4, Mux/4
  Plus1_5/1 -> Send CAN Message/6, Mux/6
  Plus1_6/1 -> Send CAN Message/7, Mux/7
  Plus1_7/1 -> Send CAN Message/8, Mux/8
  Plus1_4/1 -> Send CAN Message/5, Mux/5
  In4/1 -> Plus1_3/1
  In5/1 -> Plus1_4/1
  In1/1 -> Plus2_0/1
  In3/1 -> Plus1_2/1
  In2/1 -> Plus1_1/1
  In8/1 -> Plus1_7/1
  In6/1 -> Plus1_5/1
  In7/1 -> Plus1_6/1

== system ECO_TestLibs/TAF_CANF/Disconnected/Subsystem4 ==
  In1 : Inport
  In2 : Inport  Port=2
  In3 : Inport  Port=3
  In4 : Inport  Port=4
  In5 : Inport  Port=5
  In6 : Inport  Port=6
  In7 : Inport  Port=7
  In8 : Inport  Port=8
  Enable : EnablePort
  Plus1_{0..7} (8 alike) : $bdroot/Plus1_0
  Send Fixed-Point CAN Message : SF_CanService_Libs/Send Fixed-Point CAN Message  typeCAN=Disconnected  channel=CAN_F  mEn=off  msgInfo=TAF_CAN_new  msgIterm=CAN0x409  msgItermStore=CAN0x409  motoBit=off  flgNoFixed=off  tSample=Task_Inherit  modeCode=Parameterless
  Transmit CAN Message : CoderSF_BSW_Libs/CAN/Transmit CAN Message  channel=CAN_F  tasktimeIndex=Task_Inherit
      settings: SourceProductName=EcoCoder Blocks
  wires:
  In4/1 -> Plus1_3/1
  In5/1 -> Plus1_4/1
  In1/1 -> Plus1_0/1
  In3/1 -> Plus1_2/1
  In2/1 -> Plus1_1/1
  In8/1 -> Plus1_7/1
  In6/1 -> Plus1_5/1
  In7/1 -> Plus1_6/1
  Plus1_0/1 -> Send Fixed-Point CAN Message/1
  Plus1_1/1 -> Send Fixed-Point CAN Message/2
  Plus1_2/1 -> Send Fixed-Point CAN Message/3
  Plus1_3/1 -> Send Fixed-Point CAN Message/4
  Plus1_5/1 -> Send Fixed-Point CAN Message/6
  Plus1_6/1 -> Send Fixed-Point CAN Message/7
  Plus1_7/1 -> Send Fixed-Point CAN Message/8
  Plus1_4/1 -> Send Fixed-Point CAN Message/5
  Send Fixed-Point CAN Message/2 -> Transmit CAN Message/2
  Send Fixed-Point CAN Message/1 -> Transmit CAN Message/1
  Send Fixed-Point CAN Message/5 -> Transmit CAN Message/5
  Send Fixed-Point CAN Message/3 -> Transmit CAN Message/3
  Send Fixed-Point CAN Message/4 -> Transmit CAN Message/4

== system ECO_TestLibs/TAF_CANF/Disconnected/Subsystem8 ==
  In1 : Inport
  In2 : Inport  Port=2
  In3 : Inport  Port=3
  In4 : Inport  Port=4
  In5 : Inport  Port=5
  In6 : Inport  Port=6
  In7 : Inport  Port=7
  In8 : Inport  Port=8
  Enable : EnablePort
  Mux : Mux  Inputs=8
  Plus1_0 : $bdroot/Plus1_0
  Plus1_{1..7} (7 alike) : $bdroot/Plus2_0
  Plus2_0 : $bdroot/Plus2_0
  Send CAN Data : CoderSF_BSW_Libs/CAN/Send CAN Data  channel=CAN_F  txlen=8  txid=hex2dec('419')  frametype=Extended(29-bit ID)  showerror=off
      settings: SourceProductName=EcoCoder Blocks
  Send CAN Message : SF_CanService_Libs/Send CAN Message   typeCAN=Disconnected  channel=CAN_F  mEn=off  msgInfo=TAF_CAN_new  msgIterm=CAN0x409x  msgItermStore=CAN0x409x  motoBit=off  flgNoFixed=off  tSample=Task_Inherit  modeCode=Parameterless
  Transmit CAN Message : CoderSF_BSW_Libs/CAN/Transmit CAN Message  channel=CAN_F  tasktimeIndex=Task_Inherit
      settings: SourceProductName=EcoCoder Blocks
  wires:
  In7/1 -> Plus1_6/1
  In6/1 -> Plus1_5/1
  In8/1 -> Plus1_7/1
  In2/1 -> Plus1_1/1
  In3/1 -> Plus1_2/1
  In1/1 -> Plus2_0/1
  In5/1 -> Plus1_4/1
  In4/1 -> Plus1_3/1
  Plus1_4/1 -> Mux/5, Send CAN Message/5
  Plus1_7/1 -> Mux/8, Send CAN Message/8
  Plus1_6/1 -> Mux/7, Send CAN Message/7
  Plus1_5/1 -> Mux/6, Send CAN Message/6
  Plus1_3/1 -> Mux/4, Send CAN Message/4
  Plus1_2/1 -> Mux/3, Send CAN Message/3
  Plus1_1/1 -> Mux/2, Send CAN Message/2
  Plus2_0/1 -> Mux/1, Send CAN Message/1
  Mux/1 -> Plus1_0/1
  Plus1_0/1 -> Send CAN Data/1
  Send CAN Message/5 -> Transmit CAN Message/5
  Send CAN Message/1 -> Transmit CAN Message/1
  Send CAN Message/4 -> Transmit CAN Message/4
  Send CAN Message/2 -> Transmit CAN Message/2
  Send CAN Message/3 -> Transmit CAN Message/3

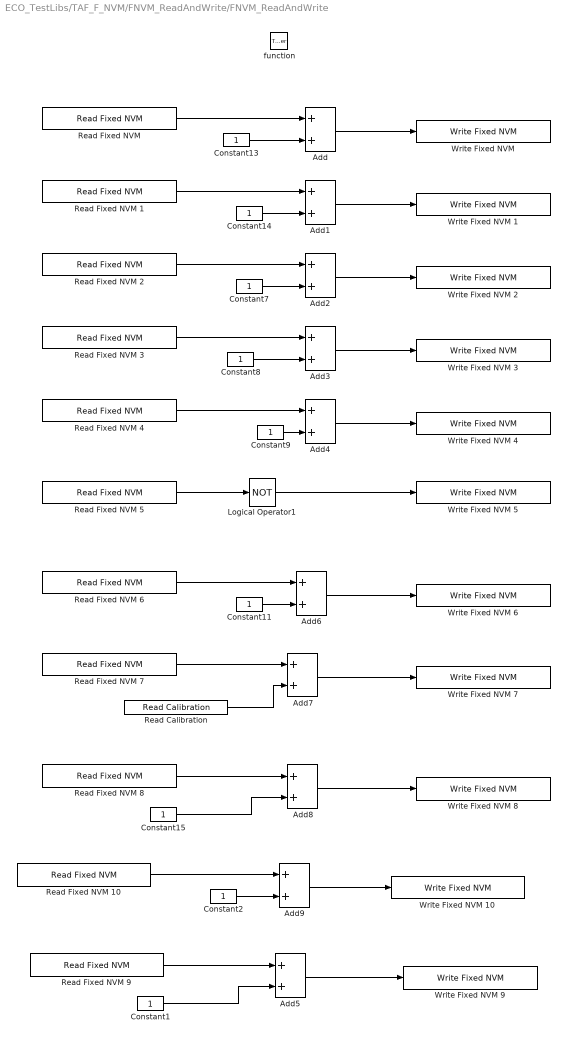
== system ECO_TestLibs/TAF_F_NVM/FNVM_ReadAndWrite/FNVM_ReadAndWrite ==
  function : TriggerPort  TriggerType=function-call  VariantControl=(inherit)
  Add{,1..9} (10 alike) : Sum  OutDataTypeStr=Inherit: Inherit via back propagation
  Constant{1..2,7..9,11,13..15} (9 alike) : Constant  OutDataTypeStr=Inherit: Inherit via back propagation  SampleTime=-1
  Logical Operator1 : Logic  Operator=NOT  AllPortsSameDT=off  OutDataTypeStr=boolean
  Read Calibration : CoderSF_BSW_Libs/Calibration & Measurement/Read Calibration  variable_name=Fnvm_int8p_VAL  variable_value=1  variable_type=int8  variable_min=[]  variable_max=[]  unitStr=""  descStr=""
      settings: AttributesFormatString=value:%<variable_value> type:%<variable_type> max:%<variable_max> Min:%<variable_min>  SourceProductName=EcoCoder Blocks
  "Read Fixed NVM " : CoderSF_BSW_Libs/Non-volatile Memory Blocks/Read Fixed NVM   data_name=Fnvm_uint32
      settings: SourceProductName=EcoCoder Blocks
  Read Fixed NVM 1 : CoderSF_BSW_Libs/Non-volatile Memory Blocks/Read Fixed NVM   data_name=Fnvm_int32
      settings: SourceProductName=EcoCoder Blocks
  Read Fixed NVM 10 : CoderSF_BSW_Libs/Non-volatile Memory Blocks/Read Fixed NVM   data_name=Fnvm_single2
      settings: SourceProductName=EcoCoder Blocks
  Read Fixed NVM 2 : CoderSF_BSW_Libs/Non-volatile Memory Blocks/Read Fixed NVM   data_name=Fnvm_single
      settings: SourceProductName=EcoCoder Blocks
  Read Fixed NVM 3 : CoderSF_BSW_Libs/Non-volatile Memory Blocks/Read Fixed NVM   data_name=Fnvm_int16
      settings: SourceProductName=EcoCoder Blocks
  Read Fixed NVM 4 : CoderSF_BSW_Libs/Non-volatile Memory Blocks/Read Fixed NVM   data_name=Fnvm_uint16
      settings: SourceProductName=EcoCoder Blocks
  Read Fixed NVM 5 : CoderSF_BSW_Libs/Non-volatile Memory Blocks/Read Fixed NVM   data_name=Fnvm_boolean
      settings: SourceProductName=EcoCoder Blocks
  Read Fixed NVM 6 : CoderSF_BSW_Libs/Non-volatile Memory Blocks/Read Fixed NVM   data_name=Fnvm_uint8
      settings: SourceProductName=EcoCoder Blocks
  Read Fixed NVM 7 : CoderSF_BSW_Libs/Non-volatile Memory Blocks/Read Fixed NVM   data_name=Fnvm_int8
      settings: SourceProductName=EcoCoder Blocks
  Read Fixed NVM 8 : CoderSF_BSW_Libs/Non-volatile Memory Blocks/Read Fixed NVM   data_name=Fnvm_double
      settings: SourceProductName=EcoCoder Blocks
  Read Fixed NVM 9 : CoderSF_BSW_Libs/Non-volatile Memory Blocks/Read Fixed NVM   data_name=Fnvm_double2
      settings: SourceProductName=EcoCoder Blocks
  "Write Fixed NVM " : CoderSF_BSW_Libs/Non-volatile Memory Blocks/Write Fixed NVM   data_name=Fnvm_uint32
      settings: SourceProductName=EcoCoder Blocks
  Write Fixed NVM 1 : CoderSF_BSW_Libs/Non-volatile Memory Blocks/Write Fixed NVM   data_name=Fnvm_int32
      settings: SourceProductName=EcoCoder Blocks
  Write Fixed NVM 10 : CoderSF_BSW_Libs/Non-volatile Memory Blocks/Write Fixed NVM   data_name=Fnvm_single2
      settings: SourceProductName=EcoCoder Blocks
  Write Fixed NVM 2 : CoderSF_BSW_Libs/Non-volatile Memory Blocks/Write Fixed NVM   data_name=Fnvm_single
      settings: SourceProductName=EcoCoder Blocks
  Write Fixed NVM 3 : CoderSF_BSW_Libs/Non-volatile Memory Blocks/Write Fixed NVM   data_name=Fnvm_int16
      settings: SourceProductName=EcoCoder Blocks
  Write Fixed NVM 4 : CoderSF_BSW_Libs/Non-volatile Memory Blocks/Write Fixed NVM   data_name=Fnvm_uint16
      settings: SourceProductName=EcoCoder Blocks
  Write Fixed NVM 5 : CoderSF_BSW_Libs/Non-volatile Memory Blocks/Write Fixed NVM   data_name=Fnvm_boolean
      settings: SourceProductName=EcoCoder Blocks
  Write Fixed NVM 6 : CoderSF_BSW_Libs/Non-volatile Memory Blocks/Write Fixed NVM   data_name=Fnvm_uint8
      settings: SourceProductName=EcoCoder Blocks
  Write Fixed NVM 7 : CoderSF_BSW_Libs/Non-volatile Memory Blocks/Write Fixed NVM   data_name=Fnvm_int8
      settings: SourceProductName=EcoCoder Blocks
  Write Fixed NVM 8 : CoderSF_BSW_Libs/Non-volatile Memory Blocks/Write Fixed NVM   data_name=Fnvm_double
      settings: SourceProductName=EcoCoder Blocks
  Write Fixed NVM 9 : CoderSF_BSW_Libs/Non-volatile Memory Blocks/Write Fixed NVM   data_name=Fnvm_double2
      settings: SourceProductName=EcoCoder Blocks
  wires:
  Logical Operator1/1 -> Write Fixed NVM 5/1
  Read Fixed NVM 5/1 -> Logical Operator1/1
  Add7/1 -> Write Fixed NVM 7/1
  Add8/1 -> Write Fixed NVM 8/1
  Constant15/1 -> Add8/2
  Read Fixed NVM 8/1 -> Add8/1
  Read Calibration/1 -> Add7/2
  Read Fixed NVM 7/1 -> Add7/1
  Constant11/1 -> Add6/2
  Read Fixed NVM 6/1 -> Add6/1
  Add6/1 -> Write Fixed NVM 6/1
  Constant9/1 -> Add4/2
  Read Fixed NVM 4/1 -> Add4/1
  Add4/1 -> Write Fixed NVM 4/1
  Constant8/1 -> Add3/2
  Read Fixed NVM 3/1 -> Add3/1
  Add3/1 -> Write Fixed NVM 3/1
  Constant7/1 -> Add2/2
  Read Fixed NVM 2/1 -> Add2/1
  Add2/1 -> Write Fixed NVM 2/1
  Constant14/1 -> Add1/2
  Read Fixed NVM 1/1 -> Add1/1
  Add1/1 -> Write Fixed NVM 1/1
  Constant13/1 -> Add/2
  "Read Fixed NVM "/1 -> Add/1
  Add/1 -> "Write Fixed NVM "/1
  Add5/1 -> Write Fixed NVM 9/1
  Constant1/1 -> Add5/2
  Read Fixed NVM 9/1 -> Add5/1
  Constant2/1 -> Add9/2
  Read Fixed NVM 10/1 -> Add9/1
  Add9/1 -> Write Fixed NVM 10/1
